simulink model "controlLaw"  (R2023b)
settings: Solver=FixedStepAuto  StartTime=0.0  StopTime=Tfinal  FixedStep=dt_cont  RelTol=1e-3
model workspace (MAT data in the model file):
  controlLaw = "dummy"
  controlType = "PD"
  dt_cont = 0.1
  errorType = "small"
  kd = [556.632039464  0  0; 0  750.755009198  0; 0  0  1152.20066554]
  kp = [17.6951093979  0  0; 0  23.8662007877  0; 0  0  36.6279972755]
libraries: rotationConversionLib x1
settings Model: Creator=kristopherriordan  LastModifiedBy=kristopherriordan

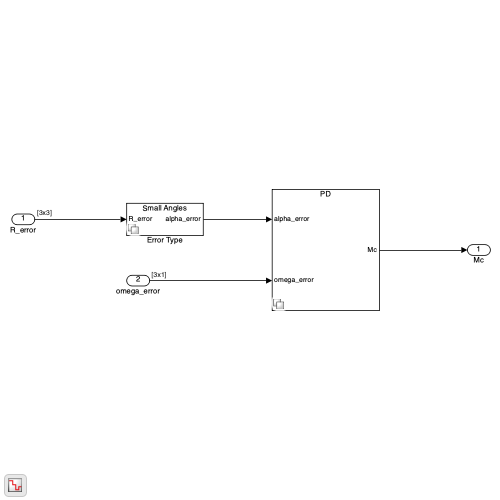
[thumbnail: Simulink's stored preview of the top-level diagram]
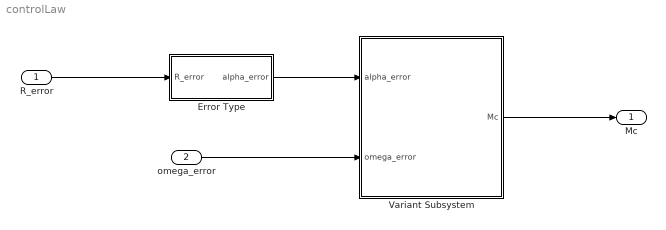
== system controlLaw ==
  R_error : Inport  PortDimensions=[3 3]
  omega_error : Inport  Port=2  PortDimensions=[3 1]
  Error Type : Subsystem  Variant=on
  Variant Subsystem : Subsystem  Variant=on
  Mc : Outport
  wires:
  Variant Subsystem/1(Mc) -> Mc/1
  omega_error/1 -> Variant Subsystem/2(omega_error)
  R_error/1 -> Error Type/1(R_error)
  Error Type/1(alpha_error) -> Variant Subsystem/1(alpha_error)

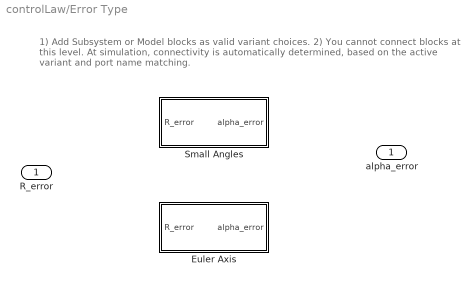
== system controlLaw/Error Type ==
  note: 1) Add Subsystem or Model blocks as valid variant choices.
      | 2) You cannot connect blocks at this level. At simulation, connectivity is automatically
      | determined, based on the active variant and port name matching.
  R_error : Inport
  "Euler Axis " : Subsystem  VariantControl="errorType==\"euler\""
  Small Angles : Subsystem  VariantControl="errorType==\"small\""
  alpha_error : Outport

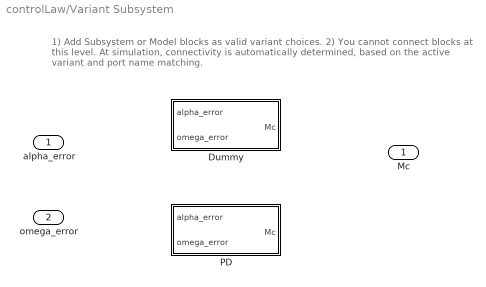
== system controlLaw/Variant Subsystem ==
  note: 1) Add Subsystem or Model blocks as valid variant choices.
      | 2) You cannot connect blocks at this level. At simulation, connectivity is automatically
      | determined, based on the active variant and port name matching.
  alpha_error : Inport
  omega_error : Inport  Port=2
  Dummy : Subsystem  VariantControl="controlType==\"dummy\""
  PD : Subsystem  VariantControl="controlType==\"PD\""
  Mc : Outport

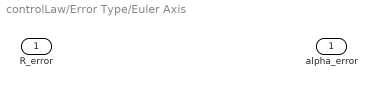
== system controlLaw/Error Type/Euler Axis  ==
  R_error : Inport
  alpha_error : Outport

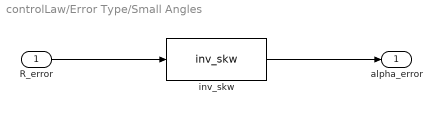
== system controlLaw/Error Type/Small Angles ==
  R_error : Inport
  inv_skw : rotationConversionLib/inv_skw  SystemSampleTime=-1  VariantActivationTime=update diagram  AllowFlexibleInterface=on  Latency=0  AutoFrameSizeCalculation=off
  alpha_error : Outport
  wires:
  R_error/1 -> inv_skw/1
  inv_skw/1 -> alpha_error/1

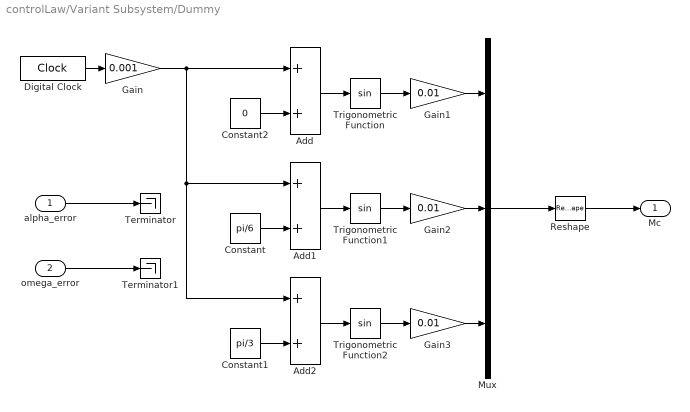
== system controlLaw/Variant Subsystem/Dummy ==
  alpha_error : Inport
  omega_error : Inport  Port=2
  Add : Sum
  Add1 : Sum
  Add2 : Sum
  Constant : Constant  Value=pi/6
  Constant1 : Constant  Value=pi/3
  Constant2 : Constant  Value=0
  Digital Clock : DigitalClock  SampleTime=dt_cont
  Gain : Gain  Gain=0.001
  Gain1 : Gain  Gain=0.01
  Gain2 : Gain  Gain=0.01
  Gain3 : Gain  Gain=0.01
  Mux : Mux  Inputs=3
  Reshape : Reshape  OutputDimensionality=Column vector (2-D)
  Terminator : Terminator
  Terminator1 : Terminator
  Trigonometric Function : Trigonometry
  Trigonometric Function1 : Trigonometry
  Trigonometric Function2 : Trigonometry
  Mc : Outport
  wires:
  alpha_error/1 -> Terminator/1
  omega_error/1 -> Terminator1/1
  Add/1 -> Trigonometric Function/1
  Add1/1 -> Trigonometric Function1/1
  Constant1/1 -> Add2/2
  Add2/1 -> Trigonometric Function2/1
  Constant/1 -> Add1/2
  Constant2/1 -> Add/2
  Gain/1 -> Add2/1, Add1/1, Add/1
  Mux/1 -> Reshape/1
  Reshape/1 -> Mc/1
  Trigonometric Function/1 -> Gain1/1
  Trigonometric Function1/1 -> Gain2/1
  Trigonometric Function2/1 -> Gain3/1
  Digital Clock/1 -> Gain/1
  Gain1/1 -> Mux/1
  Gain2/1 -> Mux/2
  Gain3/1 -> Mux/3

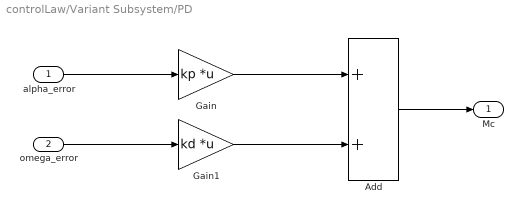
== system controlLaw/Variant Subsystem/PD ==
  alpha_error : Inport
  omega_error : Inport  Port=2
  Add : Sum
  Gain : Gain  Gain=kp  Multiplication=Matrix(K*u)
  Gain1 : Gain  Gain=kd  Multiplication=Matrix(K*u)
  Mc : Outport
  wires:
  alpha_error/1 -> Gain/1
  omega_error/1 -> Gain1/1
  Add/1 -> Mc/1
  Gain1/1 -> Add/2
  Gain/1 -> Add/1
